simulink model "p2"  (R2024a)
settings: Solver=VariableStepAuto  StartTime=0.0  StopTime=10.0  RelTol=1e-3
settings Model: Creator=Home  LastModifiedBy=Home

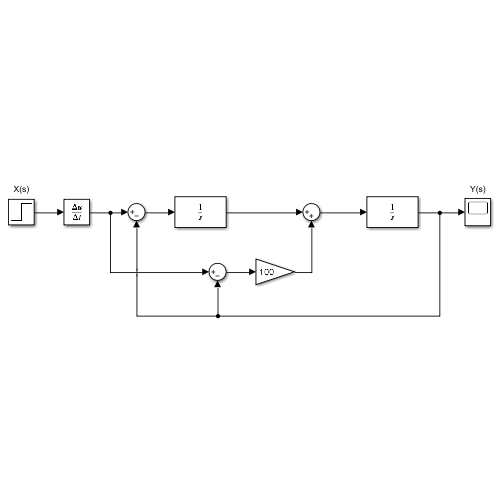
[thumbnail: Simulink's stored preview of the top-level diagram]
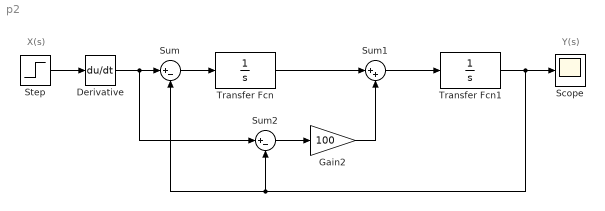
== system p2 ==
  note: X(s)
  note: Y(s)
  Derivative : Derivative
  Gain2 : Gain  Gain=100
  Scope : Scope
  Step : Step  Time=0.001  SampleTime=0
  Sum : Sum  Inputs=|+-
  Sum1 : Sum  Inputs=|++
  Sum2 : Sum  Inputs=|+-
  Transfer Fcn : TransferFcn  Denominator=[1 0]
  Transfer Fcn1 : TransferFcn  Denominator=[1 0]
  wires:
  Sum1/1 -> Transfer Fcn1/1
  Derivative/1 -> Sum2/1, Sum/1
  Sum/1 -> Transfer Fcn/1
  Transfer Fcn1/1 -> Scope/1, Sum2/2, Sum/2
  Transfer Fcn/1 -> Sum1/1
  Sum2/1 -> Gain2/1
  Gain2/1 -> Sum1/2
  Step/1 -> Derivative/1
